simulink model "IonSatSimulation"  (R2019b)
settings: Solver=VariableStepAuto  StartTime=0.0  StopTime=50000  FixedStep=10  RelTol=1e-3
model workspace (MAT data in the model file):
  Inertia = 1
undefined symbols (not defined in the file): deg, I_sat, IAU, mass, mu_Earth, rad, s
libraries: aerolibconvert2 x2, aerolibanim x1, simulink x1, shared6dof x1, aerolibtransform2 x1, aerolibgravity2 x1
settings Model: Creator=robin  LastModifiedBy=robin

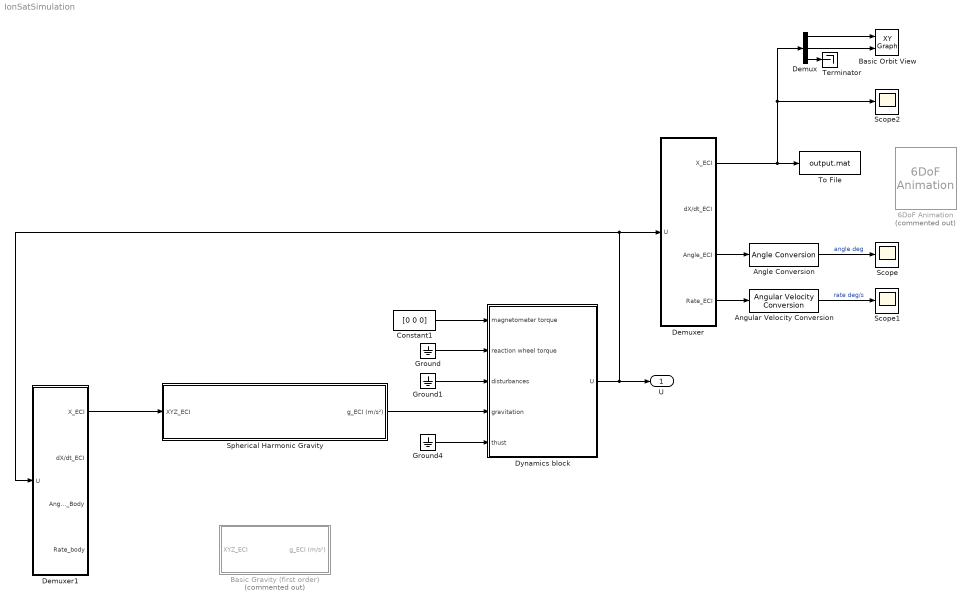
== system IonSatSimulation ==
  6DoF Animation : aerolibanim/6DoF Animation  Commented=on  u1=[-2000 2000 -2000 2000 -2000 2000]  u2=0.1  u3=1000  u4=[0 0 0]  u5=Fixed position  u6=[500 500 500]  u7=60  u8=on
      settings: SourceProductName=Aerospace Blockset
  Angle Conversion : aerolibconvert2/Angle Conversion  IU=rad  OU=deg
  Angular Velocity Conversion : aerolibconvert2/Angular Velocity Conversion  IU=rad/s  OU=deg/s
      settings: SourceProductName=Aerospace Blockset
  Basic Gravity (first order) : Subsystem  Commented=on
  Basic Orbit View : simulink/Sinks/XY Graph  xmin=-10000000  xmax=10000000  ymin=-10000000  ymax=10000000  st=-1
  Constant1 : Constant  Value=[0 0 0]
  Demux : Demux  Outputs=3
  Demuxer : Subsystem
  Demuxer1 : Subsystem
  Dynamics block : Subsystem
  Ground : Ground
  Ground1 : Ground
  Ground4 : Ground
  Scope : Scope
  Scope1 : Scope
  Scope2 : Scope
  Spherical Harmonic Gravity : Subsystem
  Terminator : Terminator
  To File : ToFile  Filename=output.mat  MatrixName=XYZ  SaveFormat=Timeseries
  U : Outport
  wires:
  Dynamics block/1(U) -> U/1, Demuxer/1(U), Demuxer1/1(U)
  Ground/1 -> Dynamics block/2(reaction wheel torque)
  Ground1/1 -> Dynamics block/3(disturbances)
  Ground4/1 -> Dynamics block/5(thust)
  Constant1/1 -> Dynamics block/1(magnetometer torque)
  Angle Conversion/1 -> Scope/1  "angle deg"
  Angular Velocity Conversion/1 -> Scope1/1  "rate deg/s"
  Demux/1 -> Basic Orbit View/1
  Demux/2 -> Basic Orbit View/2
  Demuxer/1(X_ECI) -> To File/1, Scope2/1, Demux/1
  Demux/3 -> Terminator/1
  Demuxer/4(Rate_ECI) -> Angular Velocity Conversion/1
  Demuxer/3(Angle_ECI) -> Angle Conversion/1
  Demuxer1/1(X_ECI) -> Spherical Harmonic Gravity/1(XYZ_ECI)
  Spherical Harmonic Gravity/1(g_ECI (m/s²)) -> Dynamics block/4(gravitation)

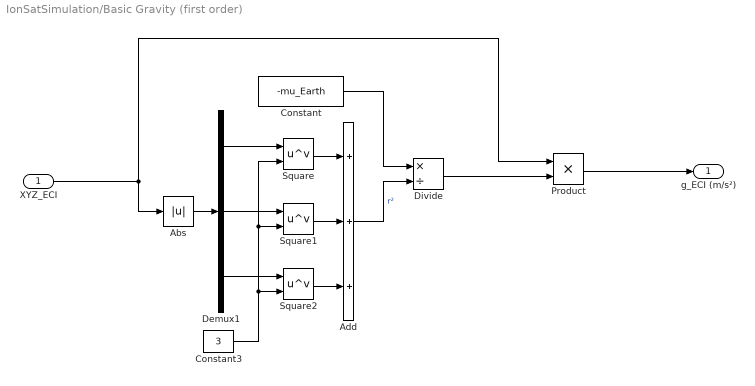
== system IonSatSimulation/Basic Gravity (first order) ==
  XYZ_ECI : Inport
  Abs : Abs
  Add : Sum  Inputs=+++
  Constant : Constant  Value=-mu_Earth
  Constant3 : Constant  Value=3
  Demux1 : Demux  Outputs=3
  Divide : Product  Inputs=*/
  Product : Product
  Square : Math  Operator=pow  SignedPower=off  SaturateOnIntegerOverflow=on
  Square1 : Math  Operator=pow  SignedPower=off  SaturateOnIntegerOverflow=on
  Square2 : Math  Operator=pow  SignedPower=off  SaturateOnIntegerOverflow=on
  g_ECI (m/s²) : Outport
  wires:
  Demux1/2 -> Square1/1
  Demux1/3 -> Square2/1
  Square/1 -> Add/1
  Square1/1 -> Add/2
  Add/1 -> Divide/2  "r²"
  Demux1/1 -> Square/1
  Square2/1 -> Add/3
  Constant/1 -> Divide/1
  Divide/1 -> Product/2
  Product/1 -> g_ECI (m/s²)/1
  Constant3/1 -> Square/2, Square1/2, Square2/2
  XYZ_ECI/1 -> Product/1, Abs/1
  Abs/1 -> Demux1/1

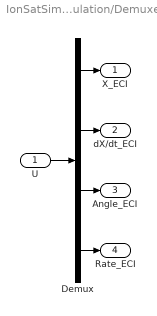
== system IonSatSimulation/Demuxer ==
  U : Inport
  Demux : Demux
  X_ECI : Outport
  dX/dt_ECI : Outport  Port=2
  Angle_ECI : Outport  Port=3
  Rate_ECI : Outport  Port=4
  wires:
  Demux/3 -> Angle_ECI/1
  Demux/1 -> X_ECI/1
  Demux/2 -> dX/dt_ECI/1
  U/1 -> Demux/1
  Demux/4 -> Rate_ECI/1

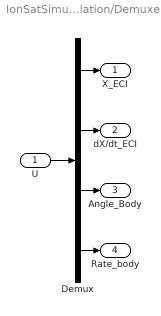
== system IonSatSimulation/Demuxer1 ==
  U : Inport
  Demux : Demux
  X_ECI : Outport
  dX/dt_ECI : Outport  Port=2
  Angle_Body : Outport  Port=3
  Rate_body : Outport  Port=4
  wires:
  Demux/3 -> Angle_Body/1
  Demux/1 -> X_ECI/1
  Demux/2 -> dX/dt_ECI/1
  U/1 -> Demux/1
  Demux/4 -> Rate_body/1

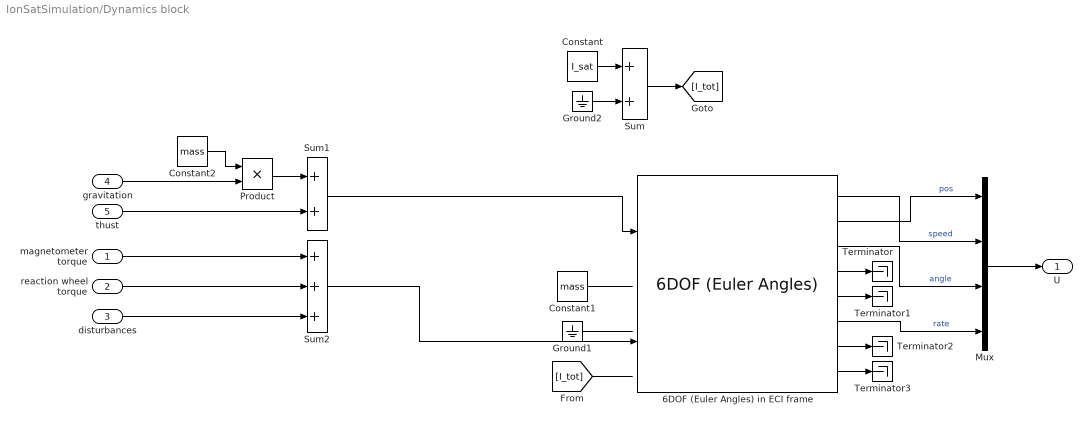
== system IonSatSimulation/Dynamics block ==
  magnetometer torque : Inport
  reaction wheel torque : Inport  Port=2  PortDimensions=3
  disturbances : Inport  Port=3  PortDimensions=3
  gravitation : Inport  Port=4  PortDimensions=3
  thust : Inport  Port=5  PortDimensions=3
  6DOF (Euler Angles) in ECI frame : shared6dof/6DOF (Euler Angles)  units=Metric (MKS)  mtype=Custom Variable  rep=Quaternion  xme_0=[7000000 0 0]  Vm_0=[0 7300 0]  eul_0=[0 0 0]  pm_0=[0 0 0]  mass_0=1.0  mass_e=0.5  mass_f=2.0  inertia=eye(3)  inertia_e=eye(3)  inertia_f=2*eye(3)  k_quat=1.0  vre_flag=off  abi_flag=off  aMode=0  xme_statename=''  Vm_statename=''  eul_statename=''  quat_statename=''  pm_statename=''  mass_statename=''
      settings: SourceProductBaseCode=AE
  Constant : Constant  Value=I_sat
  Constant1 : Constant  Value=mass
  Constant2 : Constant  Value=mass
  Ground1 : Ground
  Ground2 : Ground
  Mux : Mux
  Product : Product
  Sum : Sum
  Sum1 : Sum
  Sum2 : Sum  Inputs=+++
  Terminator{,1..3} (4 alike) : Terminator
  U : Outport  PortDimensions=12
  wires:
  6DOF (Euler Angles) in ECI frame/1 -> Mux/2  "speed"
  [I_tot] -> ?
  6DOF (Euler Angles) in ECI frame/2 -> Mux/1  "pos"
  reaction wheel torque/1 -> Sum2/2
  Ground1/1 -> ?
  disturbances/1 -> Sum2/3
  Sum1/1 -> 6DOF (Euler Angles) in ECI frame/1
  thust/1 -> Sum1/2
  magnetometer torque/1 -> Sum2/1
  Mux/1 -> U/1
  Sum2/1 -> 6DOF (Euler Angles) in ECI frame/2
  Constant1/1 -> ?
  6DOF (Euler Angles) in ECI frame/5 -> Terminator1/1
  6DOF (Euler Angles) in ECI frame/8 -> Terminator3/1
  6DOF (Euler Angles) in ECI frame/4 -> Terminator/1
  6DOF (Euler Angles) in ECI frame/7 -> Terminator2/1
  Sum/1 -> [I_tot]
  Ground2/1 -> Sum/2
  Constant/1 -> Sum/1
  6DOF (Euler Angles) in ECI frame/6 -> Mux/4  "rate"
  6DOF (Euler Angles) in ECI frame/3 -> Mux/3  "angle"
  Constant2/1 -> Product/1
  gravitation/1 -> Product/2
  Product/1 -> Sum1/1

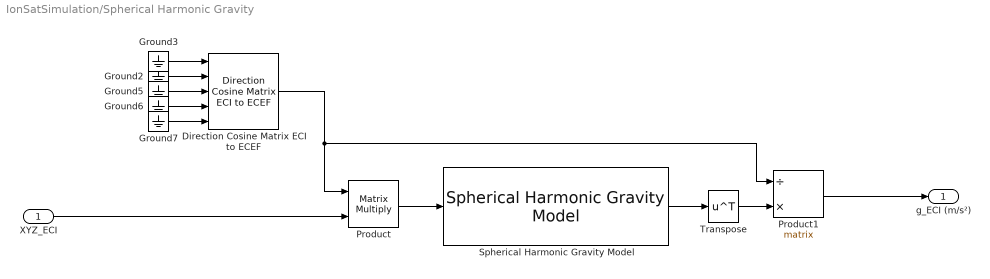
== system IonSatSimulation/Spherical Harmonic Gravity ==
  XYZ_ECI : Inport
  Direction Cosine Matrix ECI to ECEF : aerolibtransform2/Direction Cosine Matrix ECI to ECEF  red=IAU-2000/2006  year=2020  month=January  day=1  hour=0  min=0  sec=0  deltaT=Day  errorflag=Error  extraparamflag=on
      settings: AttributesFormatString=%<red>  SourceProductName=Aerospace Blockset  SourceProductBaseCode=AE
  Ground{2..3,5..7} (5 alike) : Ground
  Product : Product  Multiplication=Matrix(*)
  Product1 : Product  Inputs=/*  Multiplication=Matrix(*)
  Spherical Harmonic Gravity Model : aerolibgravity2/Spherical Harmonic Gravity Model  units=Metric (MKS)  degree=100  action=Warning  ptype=EGM2008  datafile='aerogmm2b.mat'
      settings: SourceProductName=Aerospace Blockset  SourceProductBaseCode=AE
  Transpose : Math  Operator=transpose  SignedPower=off  SaturateOnIntegerOverflow=on
  g_ECI (m/s²) : Outport
  wires:
  Ground5/1 -> Direction Cosine Matrix ECI to ECEF/3
  Direction Cosine Matrix ECI to ECEF/1 -> Product1/1, Product/1
  Transpose/1 -> Product1/2
  Ground3/1 -> Direction Cosine Matrix ECI to ECEF/1
  Ground7/1 -> Direction Cosine Matrix ECI to ECEF/5
  Ground2/1 -> Direction Cosine Matrix ECI to ECEF/2
  Product/1 -> Spherical Harmonic Gravity Model/1
  Spherical Harmonic Gravity Model/1 -> Transpose/1
  XYZ_ECI/1 -> Product/2
  Ground6/1 -> Direction Cosine Matrix ECI to ECEF/4
  Product1/1 -> g_ECI (m/s²)/1
